simulink model "test"  (R2022b)
settings: Solver=ode23tb  StartTime=0.0  StopTime=24*3600  RelTol=1e-3
libraries: ET3036TU_model_library_2021b x8, spspowerguiLib x1
settings Model: SimulationMode=accelerator  Creator=nkpanda  LastModifiedBy=jeroen
settings DebuggingCC: UnconnectedInputMsg=warning  UnconnectedOutputMsg=warning  UnconnectedLineMsg=warning
settings ModelReferenceCC: EnableRefExpFcnMdlSchedulingChecks=on
settings RTWCC: DLArmComputeVersion=19.05

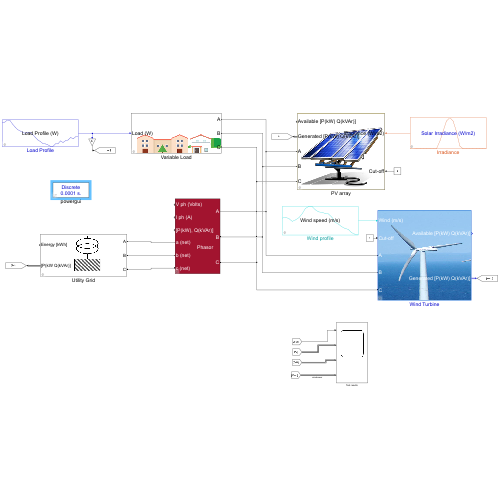
[thumbnail: Simulink's stored preview of the top-level diagram]
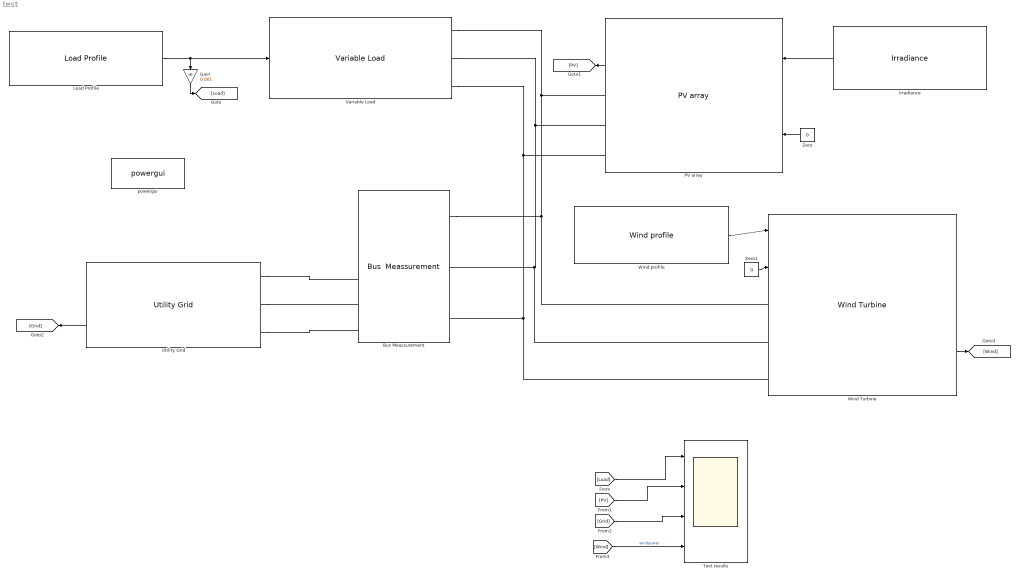
== system test ==
  "Bus Meassurement " : ET3036TU_model_library_2021b/Bus  Meassurement 
  Gain : Gain  Gain=0.001
  Irradiance : ET3036TU_model_library_2021b/Irradiance
  Load Profile : ET3036TU_model_library_2021b/Load Profile
  "PV array " : ET3036TU_model_library_2021b/PV array   Efficiency=0.2  Area=100
  Test results : Scope  NumInputPorts=4
  Utility Grid : ET3036TU_model_library_2021b/Utility Grid
      link override "Bus  Meassurement ": SourceBlock="ET3036TU_model_library_2021b/Voltage//frequency regulator/Bus  Meassurement"
  Variable Load : ET3036TU_model_library_2021b/Variable Load  PF=1  Load0=0
  "Wind Turbine " : ET3036TU_model_library_2021b/Wind Turbine     Unom=15  Umax=25  Umin=5  Pselect=1: Simple Cubic Power  Pnom=20  rp=5  Cp=16/27  rho=1.225  Uvec=1:1:30  Pvec=[0,0,0,0,21359.3750000000,58193.5000000000,104316.125000000,157104.500000000,213935.875000000,272187.500000000,329236.625000000,382460.500000000,429236.375000000,466941.500000000,492953.125000000,500000,500000,500000,500000,500000,500000,500000,500000,500000,500000,0,0,0,0,0]  Tp=1  Tq=0.1  ReactP=0
  Wind profile : ET3036TU_model_library_2021b/Wind profile
  Zero : Constant  Value=0  OutDataTypeStr=Inherit: Inherit via back propagation
  Zero1 : Constant  Value=0  OutDataTypeStr=Inherit: Inherit via back propagation
  powergui : spspowerguiLib/powergui  Priority=1  SimulationMode=Discrete  SampleTime=1e-4  frequency=Fnom  Iterations=50  frequencyindice=50  Pbase=100e6  ErrMax=1e-4  UnitsV=kV  UnitsW=MW  buscounter=0  FunctionMessages=off  echomessages=off  EnableUseOfTLC=off  CurrentSourceSwitches=off  DisableSnubberDevices=off  DisableRonSwitches=off  DisableVfSwitches=off  DisplayEquations=off  AutomaticDiscreteSolvers=off  SolverType=Tustin/Backward Euler (TBE)  Interpol=off  ExternalGateDelay=off  methode=off  Ts=100  x0status=blocks  SPID=on  SwTol=0  HookPort=off  NonlinearTolerance=1e-4  nMaxIteration=100  ContinueOnMaxIteration=off  RestoreLinks=warning  ResistiveCurrentMeasurement=off  Frange=[0:2:500]  Ylog=off  Xlog=on  ShowGrid=off  save=off  variable=ZData  structure=0  ZoomFFT=off  StartTime=0.0  cycles=1  DisplayStyle=1  fundamental=60  FreqAxis=off  MaxFrequency=1000  frequencyindicesteady=1  RmsSteady=1  display=off
  wires:
  Load Profile/1 -> Gain/1, Variable Load/1
  Irradiance/1 -> "PV array "/1
  "PV array "/2 -> [PV]
  Zero/1 -> "PV array "/2
  [PV] -> Test results/2
  Utility Grid/2 -> [Grid]
  [Grid] -> Test results/3
  Wind profile/1 -> "Wind Turbine "/1
  Zero1/1 -> "Wind Turbine "/2
  [Wind] -> Test results/4  "windpower"
  "Wind Turbine "/2 -> [Wind]
  [Load] -> Test results/1
  Gain/1 -> [Load]
  connections:
  Utility Grid/LConn1 -- "Bus Meassurement "/RConn1
  Utility Grid/LConn2 -- "Bus Meassurement "/RConn2
  Utility Grid/LConn3 -- "Bus Meassurement "/RConn3
  "PV array "/RConn2 -- "Wind Turbine "/LConn2 -- "Bus Meassurement "/LConn2 -- Variable Load/RConn2
  "Bus Meassurement "/LConn1 -- "Wind Turbine "/LConn1 -- Variable Load/RConn1 -- "PV array "/RConn1
  "PV array "/RConn3 -- "Wind Turbine "/LConn3 -- "Bus Meassurement "/LConn3 -- Variable Load/RConn3
